simulink model "RampXYSimulation"  (R2013b)
settings: Solver=ode45  StartTime=0.0  StopTime=85.71  RelTol=1e-3
libraries: simulink x1
settings Model: Creator=DEL  LastModifiedBy=DEL

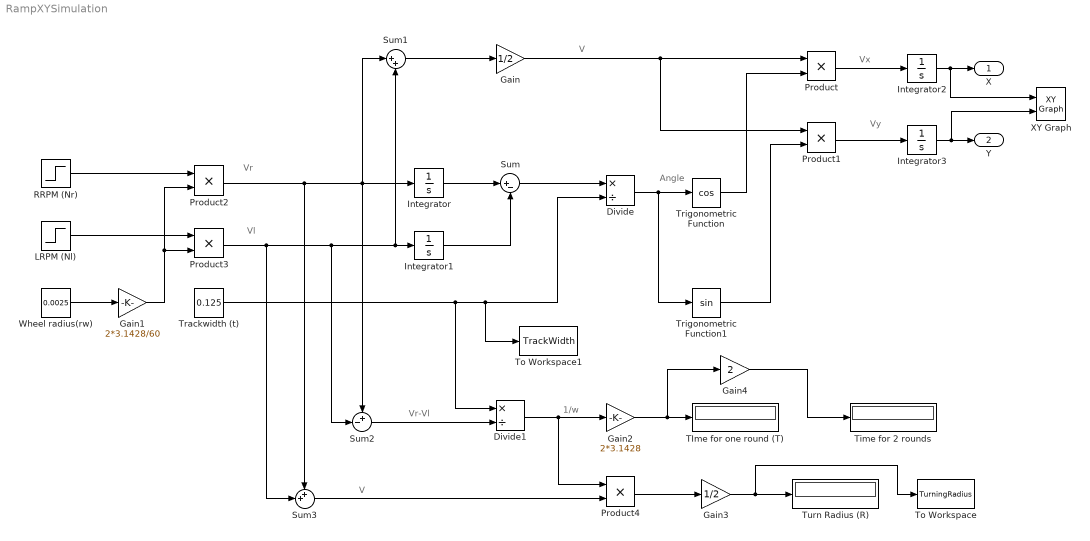
== system RampXYSimulation ==
  note: Vr-Vl
  note: V
  note: 1/w
  note: Vl
  note: Vr
  note: Vy
  note: Vx
  note: Angle
  note: V
  Divide : Product  Inputs=*/
  Divide1 : Product  Inputs=*/
  Gain : Gain  Gain=1/2
  Gain1 : Gain  Gain=2*3.1428/60
  Gain2 : Gain  Gain=2*3.1428
  Gain3 : Gain  Gain=1/2
  Gain4 : Gain  Gain=2
  Integrator{,1..3} (4 alike) : Integrator
  LRPM (Nl) : Step  Time=42.86  Before=230  After=300  SampleTime=0
  Product{,1..4} (5 alike) : Product
  RRPM (Nr) : Step  Time=42.85  Before=300  After=230  SampleTime=0
  Sum : Sum  Inputs=|+-
  Sum1 : Sum  Inputs=|++
  Sum2 : Sum  Inputs=+-|
  Sum3 : Sum  Inputs=++|
  TIme for one round (T) : Display
  Time for 2 rounds : Display
  To Workspace : ToWorkspace  VariableName=TurningRadius  SampleTime=-1
  To Workspace1 : ToWorkspace  VariableName=TrackWidth  SampleTime=-1
  Trackwidth (t) : Constant  Value=0.125
  Trigonometric Function : Trigonometry  Operator=cos
  Trigonometric Function1 : Trigonometry
  Turn Radius (R) : Display
  Wheel radius(rw) : Constant  Value=0.0025
  XY Graph : simulink/Sinks/XY Graph  xmin=-1.5  xmax=1.5  ymin=-1.5  ymax=1.5  st=-1
  X : Outport
  Y : Outport  Port=2
  wires:
  Product3/1 -> Sum3/2, Sum2/2, Sum1/2, Integrator1/1
  Integrator/1 -> Sum/1
  Integrator1/1 -> Sum/2
  Sum/1 -> Divide/1
  Trackwidth (t)/1 -> To Workspace1/1, Divide/2, Divide1/1
  Sum1/1 -> Gain/1
  Divide/1 -> Trigonometric Function/1, Trigonometric Function1/1
  Gain/1 -> Product/1, Product1/1
  Trigonometric Function/1 -> Product/2
  Trigonometric Function1/1 -> Product1/2
  Product/1 -> Integrator2/1
  Product1/1 -> Integrator3/1
  Integrator2/1 -> XY Graph/1, X/1
  Integrator3/1 -> XY Graph/2, Y/1
  RRPM (Nr)/1 -> Product2/1
  LRPM (Nl)/1 -> Product3/1
  Gain1/1 -> Product2/2, Product3/2
  Wheel radius(rw)/1 -> Gain1/1
  Gain2/1 -> Gain4/1, TIme for one round (T)/1
  Divide1/1 -> Product4/1, Gain2/1
  Product2/1 -> Sum3/1, Integrator/1, Sum2/1, Sum1/1
  Sum2/1 -> Divide1/2
  Sum3/1 -> Product4/2
  Product4/1 -> Gain3/1
  Gain3/1 -> To Workspace/1, Turn Radius (R)/1
  Gain4/1 -> Time for 2 rounds/1
